simulink subsystem "Magnitude"  (R2022a)
settings: Solver=VariableStepAuto  StartTime=0.0  StopTime=10.0  RelTol=1e-3
libraries: simulink x2
settings Model: Creator=mmarq  LastModifiedBy=mmarq

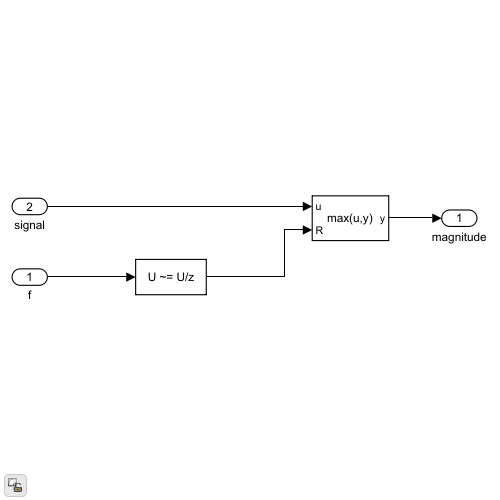
[thumbnail: Simulink's stored preview of the top-level diagram]
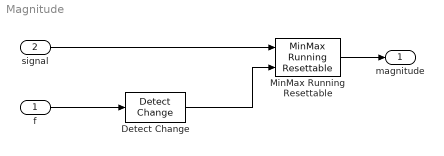
== system Magnitude ==
  f : Inport
  signal : Inport  Port=2
  Detect Change : simulink/Logic and Bit Operations/Detect Change  vinit=0  OutDataTypeStr=boolean
  MinMax Running Resettable : simulink/Math Operations/MinMax Running Resettable  Function=max  vinit=0.0
  magnitude : Outport
  wires:
  MinMax Running Resettable/1 -> magnitude/1
  f/1 -> Detect Change/1
  signal/1 -> MinMax Running Resettable/1
  Detect Change/1 -> MinMax Running Resettable/2
